simulink model "PilotSimFlex"  (Simulink 7.4)
settings: Solver=ode23tb  StartTime=0  StopTime=Inf  FixedStep=ts  MaxStep=.01  RelTol=1e-3
model workspace (MAT data in the model file):
  ts : num (value not decoded)
InitFcn:
  | if ~exist('simRunner', 'var')
  |     simRunner = PlaneRunner('simRunner');
  | end
libraries: simulink x1
settings Model: Creator=cstephen  ModifiedByFormat=Rafal  LastModifiedBy=Rafal  ExtModeArmWhenConnect=off  BufferReuse=off
settings DataIOCC: LimitDataPoints=off  SaveOutput=off  SaveTime=off  SignalLoggingName=sigsOut
settings OptimizationCC: BlockReduction=off  InlineParams=on  OptimizeBlockIOStorage=off  BufferReuse=off  EnforceIntegerDowncast=off  ExpressionFolding=off  FoldNonRolledExpr=off  LocalBlockOutputs=off  InitFltsAndDblsToZero=on
settings DebuggingCC: AlgebraicLoopMsg=none  SaveWithParameterizedLinksMsg=none  SignalResolutionControl=TryResolveAllWithWarning  SolverPrmCheckMsg=none  MultiTaskDSMMsg=warning  MultiTaskCondExecSysMsg=none  UnconnectedInputMsg=none  UnconnectedOutputMsg=none  UnconnectedLineMsg=none  StrictBusMsg=None
settings HardwareCC: TargetUnknown=on
settings RTWCC: SystemTargetFile=xpctarget.tlc  TemplateMakefile=xpc_default_tmf  ProcessScript=xpctarget_make_rtw_hook  IncludeERTFirstTime=on
settings xpcTargetCC: TargetFcnLib=ansi_tfl_tmw.mat  TargetFunctionLibrary=ANSI_C  ParMdlRefBuildCompliant=off  CompOptLevelCompliant=off  PortableWordSizes=off
settings CustomProperty: DataType=string  Value=Real-Time
settings SimMechanicsCC: VisDuringSimulation=on  VisSampleTime=0.1  LastVizWinPosition=[360 278 560 420]  CamPosition=[0;-0.208325;16.8123;]  CamTarget=[0;-0.208325;0.424625;]  CamUpVector=[0;1;0;]  CamHeight=4.41673  VisBackgroundColor=[0.9;0.9;0.95;]  DefaultBodyColor=[1;0;0;]

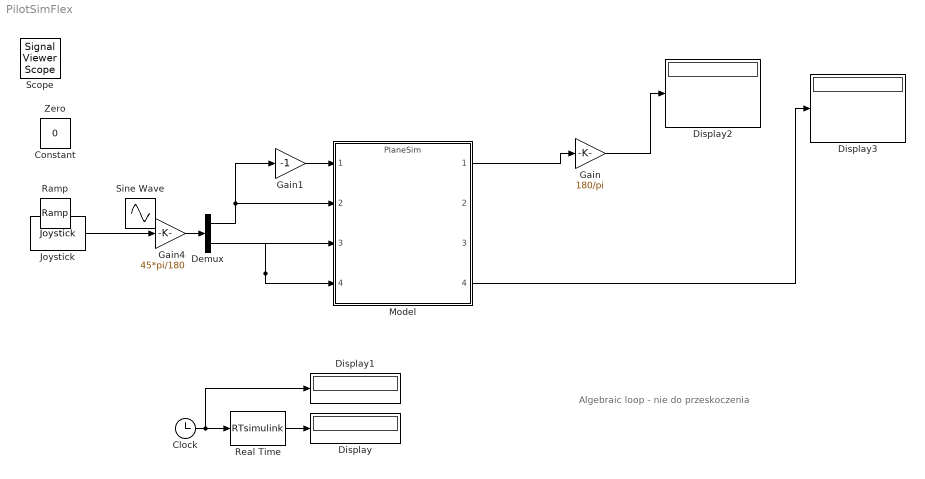
== system PilotSimFlex ==
  note: Algebraic loop - nie do przeskoczenia
  Clock : Clock
      settings: Decimation=10
  Demux : Demux  Outputs=2
  Display{,1..3} (4 alike) : Display
  Gain : Gain  Gain=180/pi  ParameterDataType=fixdt(1, 16)  ParameterScaling=2^0  OutDataType=fixdt(1, 16)  OutScaling=2^0
  Gain1 : Gain  Gain=-1  ParameterDataType=fixdt(1, 16)  ParameterScaling=2^0  OutDataType=fixdt(1, 16)  OutScaling=2^0
  Gain4 : Gain  Gain=45*pi/180  ParameterDataType=fixdt(1, 16)  ParameterScaling=2^0  OutDataType=fixdt(1, 16)  OutScaling=2^0
  Joystick : M-S-Function  FunctionName=Joystick
  Model : ModelReference  ModelNameDialog=PlaneSim  SimulationMode=Normal  ModelReferenceVersion=1.313  CopyOfModelName=PlaneSim
  Real Time : M-S-Function  FunctionName=RTsimulink
  Constant : Constant  IOType=siggen  Value=-1  OutDataType=sfix(16)  OutScaling=2^0
  Ramp : simulink/Sources/Ramp  IOType=siggen  SystemSampleTime=-1  slope=1  start=0  X0=0
  Scope : SignalViewerScope  IOType=viewer  ZoomMode=xonly  LegendLocations="674.3333      275.3333            95            41"  RefreshTime=0.035000
      settings: ShowLegends=on  YMin=-0.0018  YMax=0.0002
  Sine Wave : Sin  IOType=siggen  Amplitude=10  Bias=0  Frequency=5  Phase=pi/2  Samples=10  SampleTime=0  Offset=0
  Zero : Constant  IOType=siggen  Value=0  OutDataType=sfix(16)  OutScaling=2^0
  wires:
  Real Time/1 -> Display/1
  Clock/1 -> Display1/1, Real Time/1
  Gain4/1 -> Demux/1
  Joystick/1 -> Gain4/1
  Demux/2 -> Model/3, Model/4
  Gain1/1 -> Model/1
  Demux/1 -> Gain1/1, Model/2
  Model/1 -> Gain/1
  Gain/1 -> Display2/1
  Model/4 -> Display3/1
